simulink model "SimulinkStateflow"  (R2018a)
settings: Solver=VariableStepAuto  StartTime=0.0  StopTime=10  RelTol=1e-3
settings Model: Creator=BEAR  LastModifiedBy=BEAR

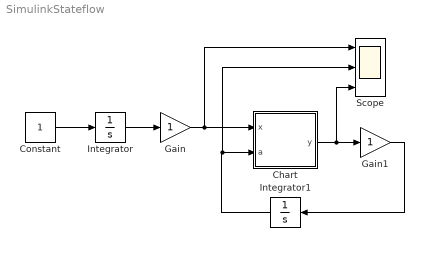
== system SimulinkStateflow ==
  Chart : Stateflow chart  TreatAsAtomicUnit=on
  Constant : Constant
  Gain : Gain  SampleTime=2
  Gain1 : Gain  SampleTime=4
  Integrator : Integrator  InitialCondition=3
  Integrator1 : Integrator  InitialCondition=2
  Scope : Scope  NumInputPorts=3
  wires:
  Constant/1 -> Integrator/1
  Integrator/1 -> Gain/1
  Gain/1 -> Scope/1, Chart/1(x)
  Chart/1(y) -> Scope/3, Gain1/1
  Gain1/1 -> Integrator1/1
  Integrator1/1 -> Scope/2, Chart/2(a)

== stateflow chart SimulinkStateflow/Chart ==
  settings: updateMethod=DISCRETE  sampleTime=3
  state on
  state off
  (default) -> on
  on -> off : {z=x+a; y = z+1}
  off -> on : {y=x-a}
  data: x input; y output; a input; z local
